simulink model "househeating_modeling"  (R2023a)
settings: Solver=VariableStepAuto  StartTime=0.0  StopTime=24  RelTol=1e-3
model workspace (MAT data in the model file):
  M_heater = 3600
  R_equivalent = 4.329e-07
  T_heater = 50
  T_roomIC = 20
  c_air = 1005.4
  m_room_air = 1474
settings Model: Creator=The MathWorks, Inc.  LastModifiedBy=oluwafemiajeigbe
settings SolverCC: AlgebraicLoopSolver=TrustRegion
settings DataIOCC: LimitDataPoints=on  SaveFormat=Array  VisualizeSimOutput=off  ReturnWorkspaceOutputs=off
settings OptimizationCC: BlockReduction=off  BooleanDataType=off  OptimizeBlockIOStorage=off  BufferReuse=off  ReuseModelBlockBuffer=off  GlobalBufferReuse=off  ExpressionFolding=off  LocalBlockOutputs=off  LifeSpan=inf
settings DebuggingCC: SaveWithParameterizedLinksMsg=none  UnderspecifiedInitializationDetection=Classic  MergeDetectMultiDrivingBlocksExec=none  SignalResolutionControl=TryResolveAllWithWarning  InheritedTsInSrcMsg=none  UnconnectedInputMsg=warning  UnconnectedOutputMsg=warning  UnconnectedLineMsg=warning  SFUnexpectedBacktrackingDiag=warning  SFNoUnconditionalDefaultTransitionDiag=warning  SFExecutionAtInitializationDiag=none  ArithmeticOperatorsInVariantConditions=warning
settings HardwareCC: ProdBitPerPointer=32  ProdBitPerSizeT=32  ProdBitPerPtrDiffT=32  ProdLargestAtomicFloat=None  ProdIntDivRoundTo=Undefined  ProdEndianess=Unspecified  ProdWordSize=32  ProdHWDeviceType=32-bit Generic  TargetUnknown=on
settings ModelReferenceCC: EnableRefExpFcnMdlSchedulingChecks=on  PropagateSignalLabelsOutOfModel=off
settings SFSimCC: SimUseLocalCustomCode=off  CustomCodeUndefinedFunction=UseInterfaceOnly
settings RTWCC: RTWUseLocalCustomCode=off
settings CodeAppCC: StateflowObjectComments=on
settings GRTTargetCC: TargetLangStandard=C89/C90 (ANSI)
settings ConfigComp: CovMetricSettings=dw  CovSaveCumulativeToWorkspaceVar=on  CovSaveSingleToWorkspaceVar=on  CovExternalEMLEnable=off  CovSFcnEnable=off

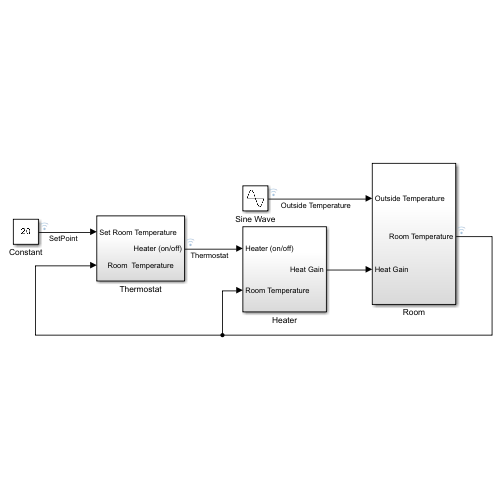
[thumbnail: Simulink's stored preview of the top-level diagram]
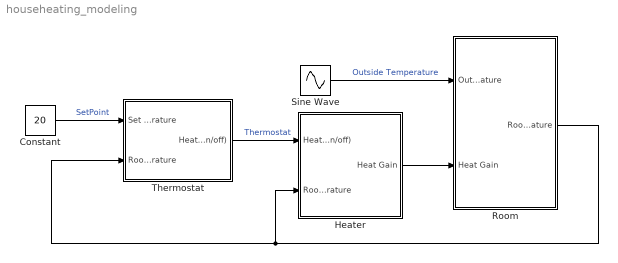
== system househeating_modeling ==
  Constant : Constant  Value=20
  Heater : Subsystem
  Room : Subsystem
  Sine Wave : Sin  Amplitude=5  Bias=19  Frequency=2*pi/24  Phase=180  SampleTime=0
  Thermostat : Subsystem
  wires:
  Thermostat/1(Heater (on/off)) -> Heater/1(Heater (on/off))  "Thermostat"
  Heater/1(Heat Gain) -> Room/2("Heat Gain ")
  Room/1(Room Temperature) -> Heater/2(Room Temperature), Thermostat/2("    Room Temperature")
  Constant/1 -> Thermostat/1(Set Room Temperature)  "SetPoint"
  Sine Wave/1 -> Room/1(Outside Temperature)  "Outside Temperature"

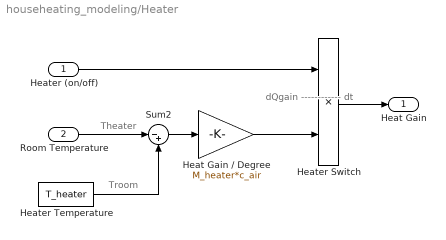
== system househeating_modeling/Heater ==
  note: dQgain
      | ------------
      |    dt
  note: Troom
  note: Theater
  Heater (on/off) : Inport
  Room Temperature : Inport  Port=2
  Heat Gain / Degree : Gain  Gain=M_heater*c_air
  Heater Switch : Product  RndMeth=Zero
  Heater Temperature : Constant  Value=T_heater
  Sum2 : Sum  Inputs=|-+
  Heat Gain : Outport  VectorParamsAs1DForOutWhenUnconnected=off
  wires:
  Heater Temperature/1 -> Sum2/2
  Room Temperature/1 -> Sum2/1
  Sum2/1 -> Heat Gain / Degree/1
  Heat Gain / Degree/1 -> Heater Switch/2
  Heater (on/off)/1 -> Heater Switch/1
  Heater Switch/1 -> Heat Gain/1

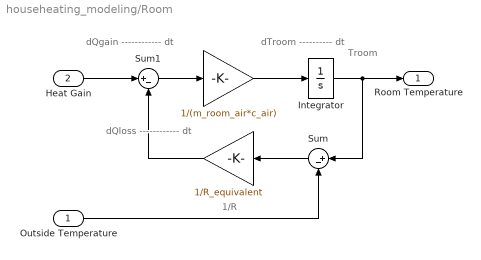
== system househeating_modeling/Room ==
  note: 1/R
  note: Troom
  note: dQloss
      | ------------
      |      dt
  note: dQgain
      | ------------
      |      dt
  note: dTroom
      | ----------
      |     dt
  Outside Temperature : Inport
  "Heat Gain " : Inport  Port=2
  " " : Gain  Gain=1/R_equivalent  SaturateOnIntegerOverflow=on  OutDataTypeStr=Inherit: Same as input  ParamDataTypeStr=Inherit: Same as input
  "  " : Gain  Gain=1/(m_room_air*c_air)  SaturateOnIntegerOverflow=on  OutDataTypeStr=Inherit: Same as input  ParamDataTypeStr=Inherit: Same as input
  Integrator : Integrator  InitialCondition=T_roomIC
  Sum : Sum  Inputs=|+-
  Sum1 : Sum  Inputs=|+-  InputSameDT=on  SaturateOnIntegerOverflow=on  OutDataTypeStr=Inherit: Same as first input
  Room Temperature : Outport  VectorParamsAs1DForOutWhenUnconnected=off
  wires:
  "Heat Gain "/1 -> Sum1/1
  Sum1/1 -> "  "/1
  "  "/1 -> Integrator/1
  Integrator/1 -> Sum/1, Room Temperature/1
  " "/1 -> Sum1/2
  Sum/1 -> " "/1
  Outside Temperature/1 -> Sum/2

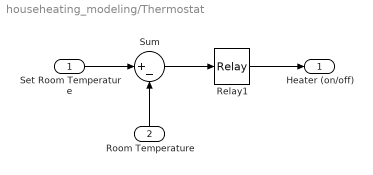
== system househeating_modeling/Thermostat ==
  Set Room Temperature : Inport
  "    Room Temperature" : Inport  Port=2
  Relay1 : Relay  OnSwitchValue=2  OffSwitchValue=-2
  Sum : Sum  Inputs=|+-  InputSameDT=on  SaturateOnIntegerOverflow=on  OutDataTypeStr=Inherit: Same as first input
  Heater (on/off) : Outport  VectorParamsAs1DForOutWhenUnconnected=off
  wires:
  Set Room Temperature/1 -> Sum/1
  Relay1/1 -> Heater (on/off)/1
  Sum/1 -> Relay1/1
  "    Room Temperature"/1 -> Sum/2
